simulink model "motorCC"  (R2020a)
settings: Solver=VariableStepAuto  StartTime=0.0  StopTime=10.0  RelTol=1e-3
values from neighbouring files (symbols this model uses):
  K = Vt_ss/(finalvalue-initialvalue)    [ganho.m]    (also in motor.mat = 0.443844062935)
  Kt = 0.0215571428571    [motor.mat]
  R = 2.3    [motor.mat]
undefined symbols (not defined in the file or in its folder): mu, Te, Tm
libraries: simulink x1
settings Model: Creator=bracj  LastModifiedBy=bracj

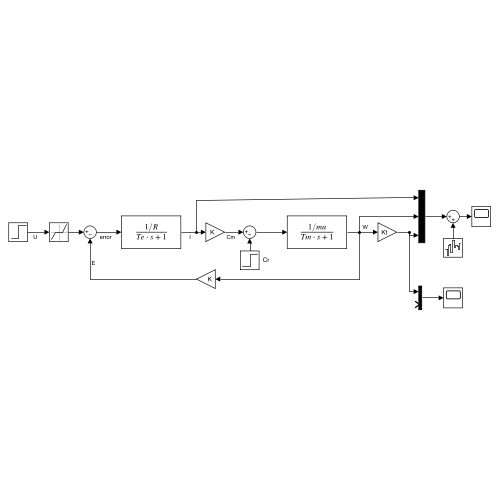
[thumbnail: Simulink's stored preview of the top-level diagram]
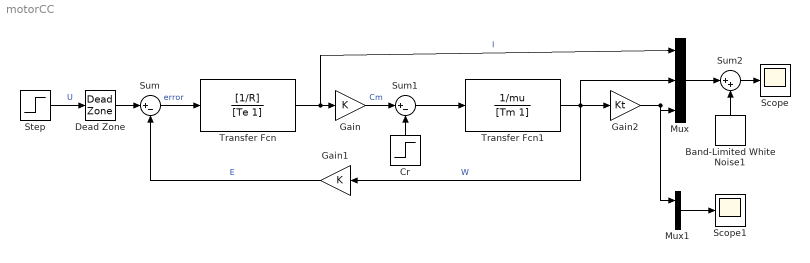
== system motorCC ==
  Band-Limited White Noise1 : simulink/Sources/Band-Limited White Noise  Cov=[0.00000001]  Ts=0.001  seed=[23341]
  Cr : Step  After=0  SampleTime=0
  Dead Zone : DeadZone  LowerValue=-3.2  UpperValue=3.2  SaturateOnIntegerOverflow=on
  Gain : Gain  Gain=K
  Gain1 : Gain  Gain=K
  Gain2 : Gain  Gain=Kt
  Mux : Mux  Inputs=3
  Mux1 : Mux  Inputs=2
  Scope : Scope
  Scope1 : Scope
  Step : Step  After=5  SampleTime=0
  Sum : Sum  Inputs=|+-
  Sum1 : Sum  Inputs=|+-
  Sum2 : Sum  Inputs=|++
  Transfer Fcn : TransferFcn  Numerator=[1/R]  Denominator=[Te 1]
  Transfer Fcn1 : TransferFcn  Numerator=1/mu  Denominator=[Tm 1]
  wires:
  Sum/1 -> Transfer Fcn/1  "error"
  Gain1/1 -> Sum/2  "E"
  Transfer Fcn/1 -> Mux/1, Gain/1  "I"
  Gain/1 -> Sum1/1  "Cm"
  Cr/1 -> Sum1/2
  Sum1/1 -> Transfer Fcn1/1
  Transfer Fcn1/1 -> Gain2/1, Mux/2, Gain1/1  "W"
  Step/1 -> Dead Zone/1  "U"
  Dead Zone/1 -> Sum/1
  Band-Limited White Noise1/1 -> Sum2/2
  Sum2/1 -> Scope/1
  Mux/1 -> Sum2/1
  Gain2/1 -> Mux1/1, Mux/3
  Mux1/1 -> Scope1/1
